simulink model "autosar_bsw_fim"  (R2022b)
settings: Solver=FixedStepAuto  StartTime=0.0  StopTime=10.0  FixedStep=0.005  RelTol=1e-3
libraries: autosarlibdem x1, autosarlibnvm x1
settings Model: Creator=The MathWorks, Inc.  LastModifiedBy=The MathWorks, Inc.
settings SolverCC: AlgebraicLoopSolver=TrustRegion  MaxZcPerStep=1
settings OptimizationCC: DefaultParameterBehavior=Inlined  EnhancedBackFolding=on  PassReuseOutputArgsAs=Individual arguments  ZeroExternalMemoryAtStartup=off  ZeroInternalMemoryAtStartup=off  OptimizeBlockOrder=speed  DifferentSizesBufferReuse=on  OptimizationCustomize=off  EfficientTunableParamExpr=on
settings DebuggingCC: ParameterTunabilityLossMsg=error  UnconnectedInputMsg=warning  UnconnectedOutputMsg=warning  UnconnectedLineMsg=warning  SFMachineParentedDataDiag=warning
settings ModelReferenceCC: EnableRefExpFcnMdlSchedulingChecks=on
settings SFSimCC: MATLABDynamicMemAlloc=off
settings RTWCC: Description=AUTOSAR  SystemTargetFile=autosar.tlc  GenCodeOnly=on  TemplateMakefile=ert_default_tmf  DLArmComputeVersion=19.05
settings CodeAppCC: ForceParamTrailComments=on  IgnoreCustomStorageClasses=off  OperatorAnnotations=on  SimulinkDataObjDesc=on  SFDataObjDesc=on  InsertBlockDesc=on
settings STFCustomTargetCC: TargetLangStandard=C99 (ISO)  MultiwordLength=256  ParMdlRefBuildCompliant=on  CompOptLevelCompliant=on  IncludeMdlTerminateFcn=off  CombineOutputUpdateFcns=on  SuppressErrorStatus=on  ERTCustomFileBanners=on  SupportNonFinite=off  SupportComplex=off  SupportContinuousTime=off  SupportNonInlinedSFcns=off  RemoveResetFunc=on  MATLABClassNameForMDSCustomization=Simulink.SoftwareTarget.ERTCustomization  AutosarCompliant=on  UseToolchainInfoCompliant=on  LookupTableObjectStructAxisOrder=2,1,3,4,...  LUTObjectStructOrderEvenSpacing=Size,Table,Breakpoints  SystemTargetFile=autosar.tlc
settings ERTTargetCC: TargetLangStandard=C99 (ISO)  ConcurrentExecutionCompliant=off  IncludeMdlTerminateFcn=off  SuppressErrorStatus=on  SupportNonFinite=off  SupportComplex=off  ModelStepFunctionPrototypeControlCompliant=off  CPPClassGenCompliant=off  AutosarCompliant=on  LookupTableObjectStructAxisOrder=2,1,3,4,...  LUTObjectStructOrderEvenSpacing=Size,Table,Breakpoints  InlinedParameterPlacement=NonHierarchical  ERTCustomFileTemplate=example_file_process.tlc

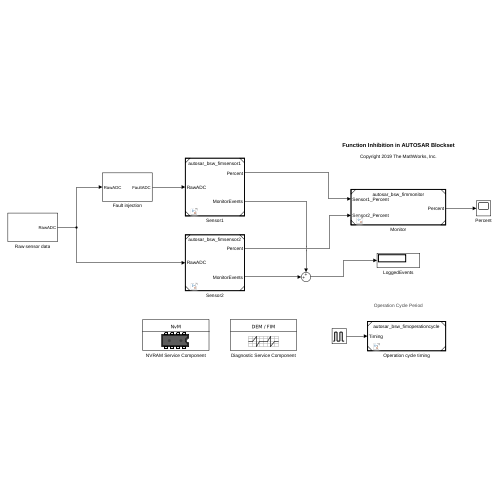
[thumbnail: Simulink's stored preview of the top-level diagram]
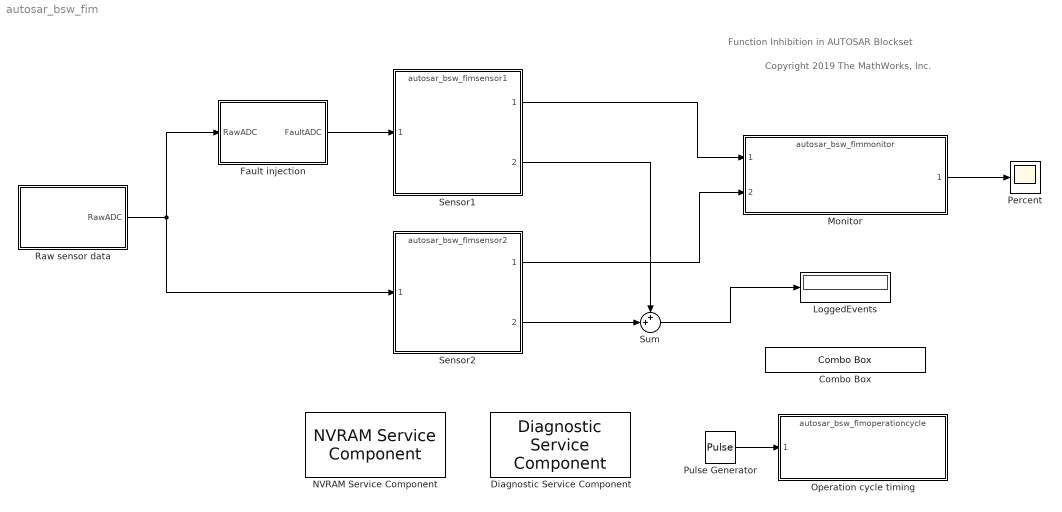
== system autosar_bsw_fim ==
  note: Copyright 2019 The MathWorks, Inc.
  note: Function Inhibition in AUTOSAR Blockset
  Combo Box : ComboBox  LabelPosition=Hide  SelectedLabel=0.1s
      settings: Values={{'0.1s', '0.3s', '0.5s', '0.8s'}, [0.1 0.3 0.5 0.8]}
      settings: AttributesFormatString=Operation Cycle Period
  Diagnostic Service Component : autosarlibdem/Diagnostic Service Component  ClientPortNames={'OperationCycle', 'S1StuckHigh', 'S1StuckLow', 'S2StuckHigh', 'S2StuckLow', 'Sensor1Valid', 'Sensor2Valid', 'TPS', 'TPSMonitor1', 'TPSMonitor2'}  ClientPortPortDefinedArguments={'1', '1', '2', '3', '4', '3', '4', '5', '1', '2'}  MaxEventId=5  MaxFID=4  DemDebounceCounterIncrementStepSize=1  DemDebounceCounterDecrementStepSize=1  DemDebounceCounterFailedThreshold=2  DemDebounceCounterPassedThreshold=-1  InhibitionMatrix=[0 0 0 0 0 0;3 3 0 0 0 0;0 0 3 3 0 0;1 1 0 0 0 0;0 0 1 1 0 0;0 0 0 0 0 0]  EnableConditionIndexes=zeros(257,'uint8')  StorageConditionIndexes=zeros(257,'uint8')
  Fault injection : Subsystem
  LoggedEvents : Display
  Monitor : ModelReference  ModelNameDialog=autosar_bsw_fimmonitor.slx  SimulationMode=Normal  ModelReferenceVersion=6.0
  NVRAM Service Component : autosarlibnvm/NVRAM Service Component  ClientPortNames={'S1LowSetPoint'}  ClientPortPortDefinedArguments={'1'}  MaxBlockId=10  NvInitValues={'0'}
  Operation cycle timing : ModelReference  ModelNameDialog=autosar_bsw_fimoperationcycle  SimulationMode=Normal  ModelReferenceVersion=6.0
  Percent : Scope
  Pulse Generator : DiscretePulseGenerator  PulseType=Time based  Period=0.1  PulseWidth=5  SampleTime=0.005
  Raw sensor data : Subsystem
  Sensor1 : ModelReference  ModelNameDialog=autosar_bsw_fimsensor1  SimulationMode=Normal  ModelReferenceVersion=6.0
  Sensor2 : ModelReference  ModelNameDialog=autosar_bsw_fimsensor2  SimulationMode=Normal  ModelReferenceVersion=6.0
  Sum : Sum  Inputs=++|
  wires:
  Raw sensor data/1(RawADC) -> Sensor2/1, Fault injection/1(RawADC)
  Monitor/1 -> Percent/1
  Sensor1/1 -> Monitor/1
  Sensor2/1 -> Monitor/2
  Fault injection/1(FaultADC) -> Sensor1/1
  Pulse Generator/1 -> Operation cycle timing/1
  Sensor1/2 -> Sum/1
  Sensor2/2 -> Sum/2
  Sum/1 -> LoggedEvents/1

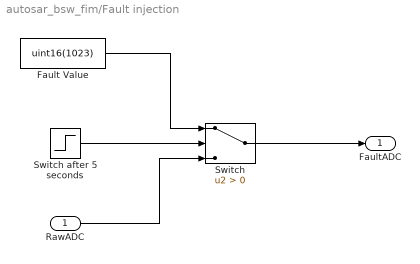
== system autosar_bsw_fim/Fault injection ==
  RawADC : Inport
  Fault Value : Constant  Value=uint16(1023)
  Switch : Switch  Criteria=u2 > Threshold  SaturateOnIntegerOverflow=off  InputSameDT=off
  Switch after 5 seconds : Step  Time=5  SampleTime=0
  FaultADC : Outport
  wires:
  RawADC/1 -> Switch/3
  Switch after 5 seconds/1 -> Switch/2
  Fault Value/1 -> Switch/1
  Switch/1 -> FaultADC/1

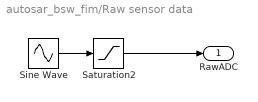
== system autosar_bsw_fim/Raw sensor data ==
  Saturation2 : Saturate  UpperLimit=1023  LowerLimit=0  LinearizeAsGain=off  ZeroCross=off  OutDataTypeStr=uint16
  Sine Wave : Sin  Amplitude=500  Frequency=3  SampleTime=0.005
  RawADC : Outport
  wires:
  Sine Wave/1 -> Saturation2/1
  Saturation2/1 -> RawADC/1
